simulink library "Rotation2D"  (R2023a)
settings: Solver=VariableStepAuto  StartTime=0.0  StopTime=10.0  RelTol=1e-3
libraries: $bdroot x1
settings Model: Creator=FIRSTMentor  LastModifiedBy=FIRSTMentor

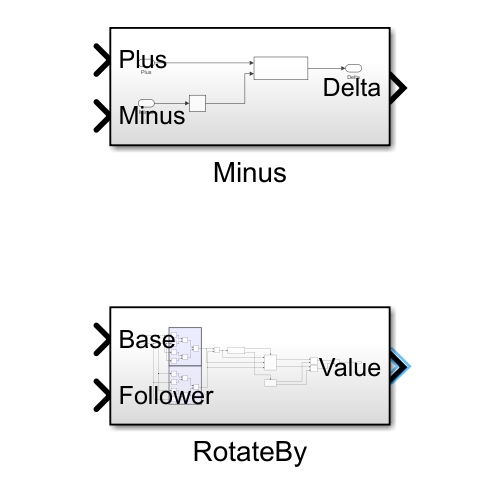
[thumbnail: Simulink's stored preview of the top-level diagram]
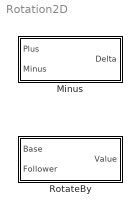
== system Rotation2D ==
  Minus : Subsystem
  RotateBy : Subsystem

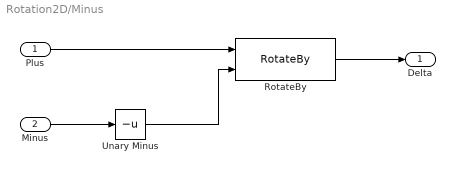
== system Rotation2D/Minus ==
  Plus : Inport
  Minus : Inport  Port=2
  RotateBy : $bdroot/RotateBy  SystemSampleTime=-1  VariantActivationTime=update diagram  Latency=0  AutoFrameSizeCalculation=off
  Unary Minus : UnaryMinus
  Delta : Outport
  wires:
  Plus/1 -> RotateBy/1
  RotateBy/1 -> Delta/1
  Minus/1 -> Unary Minus/1
  Unary Minus/1 -> RotateBy/2

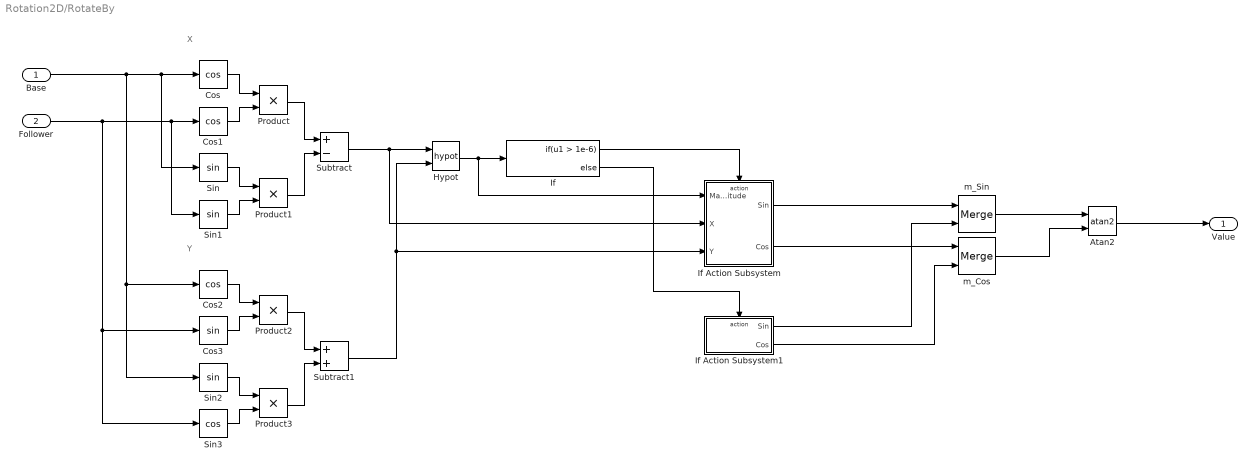
== system Rotation2D/RotateBy ==
  note: Y
  note: X
  Base : Inport  OutDataTypeStr=double  Unit=rad
  Follower : Inport  Port=2  OutDataTypeStr=double  Unit=rad
  Atan2 : Trigonometry  Operator=atan2
  Cos : Trigonometry  Operator=cos
  Cos1 : Trigonometry  Operator=cos
  Cos2 : Trigonometry  Operator=cos
  Cos3 : Trigonometry
  Hypot : Math  Operator=hypot
  If : If  IfExpression=u1 > 1e-6
  If Action Subsystem : Subsystem  TreatAsAtomicUnit=on
  If Action Subsystem1 : Subsystem  AncestorBlock=Rotation2D/RotateBy/If Action Subsystem  TreatAsAtomicUnit=on
      settings: LibrarySourceBlock=|
      | Rotation2D/RotateBy/If Action
      | Subsystem
  Product{,1..3} (4 alike) : Product
  Sin : Trigonometry
  Sin1 : Trigonometry
  Sin2 : Trigonometry
  Sin3 : Trigonometry  Operator=cos
  Subtract : Sum  Inputs=+-
  Subtract1 : Sum
  m_Cos : Merge
  m_Sin : Merge
  Value : Outport  OutDataTypeStr=double  Unit=rad
  wires:
  Base/1 -> Sin2/1, Cos2/1, Sin/1, Cos/1
  Follower/1 -> Sin3/1, Cos3/1, Sin1/1, Cos1/1
  Cos/1 -> Product/1
  Cos1/1 -> Product/2
  Sin/1 -> Product1/1
  Sin1/1 -> Product1/2
  Product/1 -> Subtract/1
  Product1/1 -> Subtract/2
  Cos3/1 -> Product2/2
  Sin3/1 -> Product3/2
  Product2/1 -> Subtract1/1
  Cos2/1 -> Product2/1
  Product3/1 -> Subtract1/2
  Sin2/1 -> Product3/1
  Atan2/1 -> Value/1
  Subtract/1 -> If Action Subsystem/2(X), Hypot/1
  Subtract1/1 -> If Action Subsystem/3(Y), Hypot/2
  Hypot/1 -> If Action Subsystem/1(Magnitude), If/1
  m_Sin/1 -> Atan2/1
  m_Cos/1 -> Atan2/2
  If/1 -> If Action Subsystem/Action
  If/2 -> If Action Subsystem1/Action
  If Action Subsystem/1(Sin) -> m_Sin/1
  If Action Subsystem1/1(Sin) -> m_Sin/2
  If Action Subsystem/2(Cos) -> m_Cos/1
  If Action Subsystem1/2(Cos) -> m_Cos/2

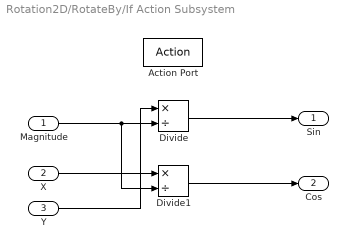
== system Rotation2D/RotateBy/If Action Subsystem ==
  Magnitude : Inport
  X : Inport  Port=2
  Y : Inport  Port=3
  Action Port : ActionPort  ActionPortLabel=if(u1 < 1e-6)
  Divide : Product  Inputs=*/
  Divide1 : Product  Inputs=*/
  Sin : Outport
  Cos : Outport  Port=2
  wires:
  Divide1/1 -> Cos/1
  Divide/1 -> Sin/1
  Magnitude/1 -> Divide1/2, Divide/2
  X/1 -> Divide1/1
  Y/1 -> Divide/1

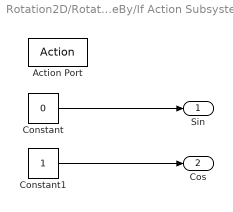
== system Rotation2D/RotateBy/If Action Subsystem1 ==
  Action Port : ActionPort
  Constant : Constant  Value=0
  Constant1 : Constant
  Sin : Outport
  Cos : Outport  Port=2
  wires:
  Constant/1 -> Sin/1
  Constant1/1 -> Cos/1
